simulink model "lab_exercice2"  (R2016a)
settings: Solver=ode3  StartTime=0.0  StopTime=0.025  FixedStep=1/100000  RelTol=1e-3
libraries: dsparch4 x1
settings Model: Creator=beac2832  LastModifiedBy=beac2832

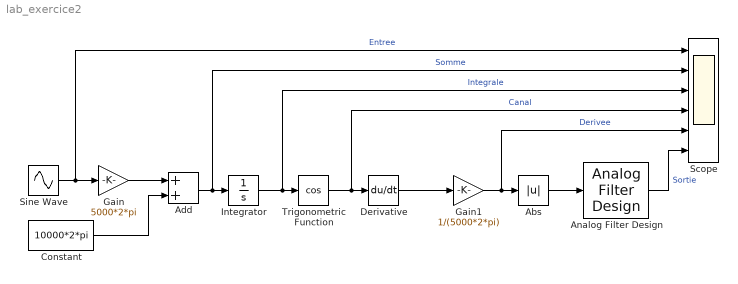
== system lab_exercice2 ==
  Abs : Abs
  Add : Sum
  Analog Filter Design : dsparch4/Analog Filter Design  method=Butterworth  filttype=Bandpass  N=2  Wlo=100*2*pi  Whi=1000*2*pi  Rp=2  Rs=40
  Constant : Constant  Value=10000*2*pi
  Derivative : Derivative
  Gain : Gain  Gain=5000*2*pi
  Gain1 : Gain  Gain=1/(5000*2*pi)
  Integrator : Integrator
  Scope : Scope  NumInputPorts=6
  Sine Wave : Sin  Frequency=200*2*pi  SampleTime=0
  Trigonometric Function : Trigonometry  Operator=cos
  wires:
  Sine Wave/1 -> Scope/1, Gain/1  "Entree"
  Gain/1 -> Add/1
  Constant/1 -> Add/2
  Add/1 -> Scope/2, Integrator/1  "Somme"
  Integrator/1 -> Scope/3, Trigonometric Function/1  "Integrale"
  Trigonometric Function/1 -> Scope/4, Derivative/1  "Canal"
  Derivative/1 -> Gain1/1
  Gain1/1 -> Scope/5, Abs/1  "Derivee"
  Abs/1 -> Analog Filter Design/1
  Analog Filter Design/1 -> Scope/6  "Sortie"
